simulink model "modelisation"  (R2018a)
settings: Solver=VariableStepAuto  StartTime=0.0  StopTime=10  RelTol=1e-3
values from neighbouring files (symbols this model uses):
  coderResolution = 370.0    (= 370)    [simu.m]
  D = xD + yD * 1i    [simu.m]
  dDirEcartMax = 5.0    (= 5)    [simu.m]
  dDirEcartMin = 1.0    (= 1)    [simu.m]
  distanceBetweenWheels = width    (= 250)    [simu.m]
  I = 0.0    (= 0)    [simu.m]
  motorNominalTension = 24.0    (= 24)    [simu.m]
  motorSpeedGain = (motorSpeedGainRPMpV / 60.0)    (= 3.88333333333)    [simu.m]
  oDirEcartMax = (45.0 / 360.0 * 2.0 * pi)    (= 0.785398163397)    [simu.m]
  oDirEcartMin = (6.0 / 360.0 * 2.0 * pi)    (= 0.10471975512)    [simu.m]
  oGain = 3.0    (= 3)    [simu.m]
  oinit = 4 * pi    (= 12.5663706144)    [simu.m]
  P = 3.0    (= 3)    [simu.m]
  reducRatio = (cranReducIn / cranReducOut)    (= 0.25)    [simu.m]
  wheelPerimeter = (wheelDiameter * pi)    (= 251.327412287)    [simu.m]
  xinit = 50    [simu.m]
  yinit = 50    [simu.m]
libraries: simulink x2
settings Model: Creator=geoffrey  LastModifiedBy=geoffrey
settings CodeAppCC: StateflowObjectComments=on

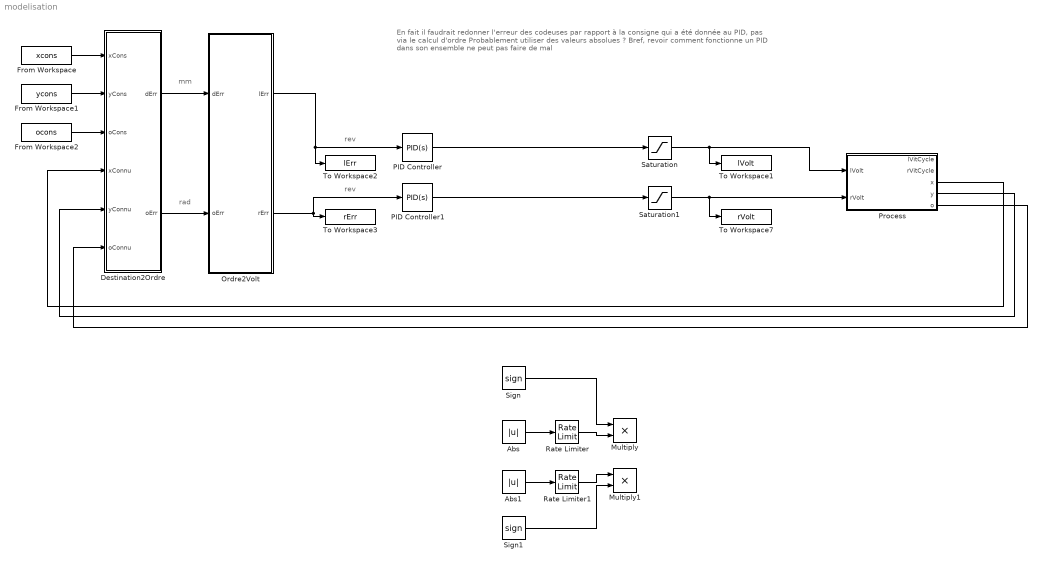
== system modelisation ==
  note: rev
  note: rad
  note: mm
  note: En fait il faudrait redonner l'erreur des codeuses par rapport à la consigne qui a été donnée au PID, pas via le calcul d'ordre
      | Probablement utiliser des valeurs absolues ?
      | Bref, revoir comment fonctionne un PID dans son ensemble ne peut pas faire de mal
  note: rev
  Abs : Abs
  Abs1 : Abs
  Destination2Ordre : Subsystem
  From Workspace : FromWorkspace  VariableName=xcons  SampleTime=0
  From Workspace1 : FromWorkspace  VariableName=ycons  SampleTime=0
  From Workspace2 : FromWorkspace  VariableName=ocons  SampleTime=0
  Multiply : Product
  Multiply1 : Product
  Ordre2Volt : Subsystem
  PID Controller : simulink/Continuous/PID Controller  Controller=PID  TimeDomain=Continuous-time  SampleTime=-1  IntegratorMethod=Forward Euler  FilterMethod=Forward Euler  Form=Parallel  UseFilter=on  ControllerParametersSource=internal  P=P  I=I  D=D  N=100  InitialConditionSource=internal  InitialConditionForIntegrator=0  InitialConditionForFilter=0  ExternalReset=none  LimitOutput=off  UpperSaturationLimit=inf  LowerSaturationLimit=-inf  LinearizeAsGain=on  AntiWindupMode=none  Kb=1  TrackingMode=off  Kt=1  PParamMin=[]  PParamMax=[]  IParamMin=[]  IParamMax=[]  DParamMin=[]  DParamMax=[]  NParamMin=[]  NParamMax=[]  KbParamMin=[]  KbParamMax=[]  KtParamMin=[]  KtParamMax=[]  POutMin=[]  POutMax=[]  IOutMin=[]  IOutMax=[]  DOutMin=[]  DOutMax=[]  NOutMin=[]  NOutMax=[]  KbOutMin=[]  KbOutMax=[]  KtOutMin=[]  KtOutMax=[]  IntegratorOutMin=[]  IntegratorOutMax=[]  FilterOutMin=[]  FilterOutMax=[]  SumOutMin=[]  SumOutMax=[]  SumI1OutMin=[]  SumI1OutMax=[]  SumI2OutMin=[]  SumI2OutMax=[]  SumI3OutMin=[]  SumI3OutMax=[]  SumDOutMin=[]  SumDOutMax=[]  SaturationOutMin=[]  SaturationOutMax=[]  IntegratorContinuousStateAttributes=''  IntegratorStateMustResolveToSignalObject=off  IntegratorRTWStateStorageClass=Auto  FilterContinuousStateAttributes=''  FilterStateMustResolveToSignalObject=off  FilterRTWStateStorageClass=Auto  DifferentiatorICPrevScaledInput=0  DifferentiatorOutMin=[]  DifferentiatorOutMax=[]  InitialConditionSetting=State (most efficient)  FilterDiffOutCoefMin=[]  FilterDiffOutCoefMax=[]  SumDenOutMin=[]  SumDenOutMax=[]  SumNumOutMin=[]  SumNumOutMax=[]  ReciprocalOutMin=[]  ReciprocalOutMax=[]  DivideOutMin=[]  DivideOutMax=[]  TunerSelectOption=Transfer Function Based (PID Tuner App)
  PID Controller1 : simulink/Continuous/PID Controller  Controller=PID  TimeDomain=Continuous-time  SampleTime=-1  IntegratorMethod=Forward Euler  FilterMethod=Forward Euler  Form=Parallel  UseFilter=on  ControllerParametersSource=internal  P=P  I=I  D=D  N=100  InitialConditionSource=internal  InitialConditionForIntegrator=0  InitialConditionForFilter=0  ExternalReset=none  LimitOutput=off  UpperSaturationLimit=inf  LowerSaturationLimit=-inf  LinearizeAsGain=on  AntiWindupMode=none  Kb=1  TrackingMode=off  Kt=1  PParamMin=[]  PParamMax=[]  IParamMin=[]  IParamMax=[]  DParamMin=[]  DParamMax=[]  NParamMin=[]  NParamMax=[]  KbParamMin=[]  KbParamMax=[]  KtParamMin=[]  KtParamMax=[]  POutMin=[]  POutMax=[]  IOutMin=[]  IOutMax=[]  DOutMin=[]  DOutMax=[]  NOutMin=[]  NOutMax=[]  KbOutMin=[]  KbOutMax=[]  KtOutMin=[]  KtOutMax=[]  IntegratorOutMin=[]  IntegratorOutMax=[]  FilterOutMin=[]  FilterOutMax=[]  SumOutMin=[]  SumOutMax=[]  SumI1OutMin=[]  SumI1OutMax=[]  SumI2OutMin=[]  SumI2OutMax=[]  SumI3OutMin=[]  SumI3OutMax=[]  SumDOutMin=[]  SumDOutMax=[]  SaturationOutMin=[]  SaturationOutMax=[]  IntegratorContinuousStateAttributes=''  IntegratorStateMustResolveToSignalObject=off  IntegratorRTWStateStorageClass=Auto  FilterContinuousStateAttributes=''  FilterStateMustResolveToSignalObject=off  FilterRTWStateStorageClass=Auto  DifferentiatorICPrevScaledInput=0  DifferentiatorOutMin=[]  DifferentiatorOutMax=[]  InitialConditionSetting=State (most efficient)  FilterDiffOutCoefMin=[]  FilterDiffOutCoefMax=[]  SumDenOutMin=[]  SumDenOutMax=[]  SumNumOutMin=[]  SumNumOutMax=[]  ReciprocalOutMin=[]  ReciprocalOutMax=[]  DivideOutMin=[]  DivideOutMax=[]  TunerSelectOption=Transfer Function Based (PID Tuner App)
  Process : Subsystem
  Rate Limiter : RateLimiter  FallingSlewLimit=-inf  SampleTimeMode=inherited
  Rate Limiter1 : RateLimiter  FallingSlewLimit=-inf  SampleTimeMode=inherited
  Saturation : Saturate  UpperLimit=motorNominalTension  LowerLimit=-motorNominalTension
  Saturation1 : Saturate  UpperLimit=motorNominalTension  LowerLimit=-motorNominalTension
  Sign : Signum
  Sign1 : Signum
  To Workspace1 : ToWorkspace  VariableName=lVolt  SaveFormat=Timeseries  SampleTime=-1
  To Workspace2 : ToWorkspace  VariableName=lErr  SaveFormat=Timeseries  SampleTime=-1
  To Workspace3 : ToWorkspace  VariableName=rErr  SaveFormat=Timeseries  SampleTime=-1
  To Workspace7 : ToWorkspace  VariableName=rVolt  SaveFormat=Timeseries  SampleTime=-1
  wires:
  Process/3(x) -> Destination2Ordre/4(xConnu)
  Process/4(y) -> Destination2Ordre/5(yConnu)
  Process/5(o) -> Destination2Ordre/6(oConnu)
  Saturation/1 -> To Workspace1/1, Process/1(lVolt)
  Saturation1/1 -> To Workspace7/1, Process/2(rVolt)
  From Workspace1/1 -> Destination2Ordre/2(yCons)
  From Workspace/1 -> Destination2Ordre/1(xCons)
  From Workspace2/1 -> Destination2Ordre/3(oCons)
  Ordre2Volt/1(lErr) -> To Workspace2/1, PID Controller/1
  Ordre2Volt/2(rErr) -> To Workspace3/1, PID Controller1/1
  Destination2Ordre/1(dErr) -> Ordre2Volt/1(dErr)
  Destination2Ordre/2(oErr) -> Ordre2Volt/2(oErr)
  PID Controller/1 -> Saturation/1
  PID Controller1/1 -> Saturation1/1
  Abs1/1 -> Rate Limiter1/1
  Sign1/1 -> Multiply1/2
  Rate Limiter/1 -> Multiply/2
  Rate Limiter1/1 -> Multiply1/1
  Abs/1 -> Rate Limiter/1
  ? -> Sign/1, Abs/1
  Sign/1 -> Multiply/1
  ? -> Sign1/1, Abs1/1

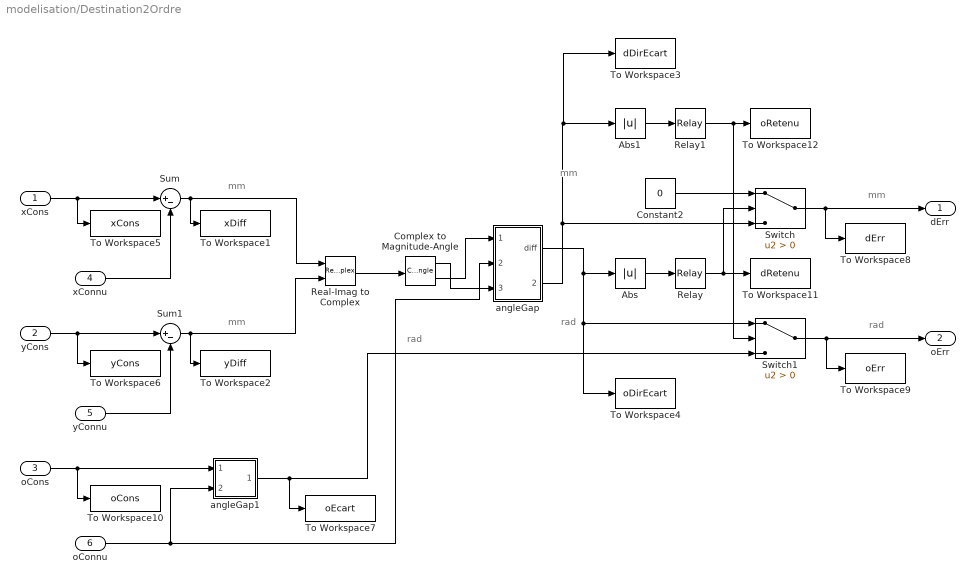
== system modelisation/Destination2Ordre ==
  note: mm
  note: rad
  note: rad
  note: mm
  note: rad
  note: mm
  note: mm
  xCons : Inport
  yCons : Inport  Port=2
  oCons : Inport  Port=3
  xConnu : Inport  Port=4
  yConnu : Inport  Port=5
  oConnu : Inport  Port=6
  Abs : Abs
  Abs1 : Abs
  Complex to Magnitude-Angle : ComplexToMagnitudeAngle
  Constant2 : Constant  Value=0
  Real-Imag to Complex : RealImagToComplex
  Relay : Relay  OnSwitchValue=oDirEcartMax  OffSwitchValue=oDirEcartMin
  Relay1 : Relay  OnSwitchValue=dDirEcartMax  OffSwitchValue=dDirEcartMin
  Sum : Sum  Inputs=|+-
  Sum1 : Sum  Inputs=|+-
  Switch : Switch  Criteria=u2 > Threshold
  Switch1 : Switch  Criteria=u2 > Threshold
  To Workspace1 : ToWorkspace  VariableName=xDiff  SaveFormat=Timeseries  SampleTime=-1
  To Workspace10 : ToWorkspace  VariableName=oCons  SaveFormat=Timeseries  SampleTime=-1
  To Workspace11 : ToWorkspace  VariableName=dRetenu  SaveFormat=Timeseries  SampleTime=-1
  To Workspace12 : ToWorkspace  VariableName=oRetenu  SaveFormat=Timeseries  SampleTime=-1
  To Workspace2 : ToWorkspace  VariableName=yDiff  SaveFormat=Timeseries  SampleTime=-1
  To Workspace3 : ToWorkspace  VariableName=dDirEcart  SaveFormat=Timeseries  SampleTime=-1
  To Workspace4 : ToWorkspace  VariableName=oDirEcart  SaveFormat=Timeseries  SampleTime=-1
  To Workspace5 : ToWorkspace  VariableName=xCons  SaveFormat=Timeseries  SampleTime=-1
  To Workspace6 : ToWorkspace  VariableName=yCons  SaveFormat=Timeseries  SampleTime=-1
  To Workspace7 : ToWorkspace  VariableName=oEcart  SaveFormat=Timeseries  SampleTime=-1
  To Workspace8 : ToWorkspace  VariableName=dErr  SaveFormat=Timeseries  SampleTime=-1
  To Workspace9 : ToWorkspace  VariableName=oErr  SaveFormat=Timeseries  SampleTime=-1
  angleGap : Subsystem
  angleGap1 : Subsystem
  dErr : Outport
  oErr : Outport  Port=2
  wires:
  xConnu/1 -> Sum/2
  xCons/1 -> Sum/1, To Workspace5/1
  Sum/1 -> Real-Imag to Complex/1, To Workspace1/1
  Sum1/1 -> Real-Imag to Complex/2, To Workspace2/1
  yConnu/1 -> Sum1/2
  Switch1/1 -> oErr/1, To Workspace9/1
  Switch/1 -> dErr/1, To Workspace8/1
  Real-Imag to Complex/1 -> Complex to Magnitude-Angle/1
  Relay/1 -> To Workspace11/1, Switch/2
  Constant2/1 -> Switch/1
  Relay1/1 -> To Workspace12/1, Switch1/2
  oConnu/1 -> angleGap1/2(actual), angleGap/2(actual)
  yCons/1 -> To Workspace6/1, Sum1/1
  oCons/1 -> angleGap1/1(target), To Workspace10/1
  Complex to Magnitude-Angle/2 -> angleGap/1(target)
  Abs/1 -> Relay/1
  angleGap/1(diff) -> Switch1/1, To Workspace4/1, Abs/1
  angleGap1/1(diff) -> To Workspace7/1, Switch1/3
  Complex to Magnitude-Angle/1 -> angleGap/3(dist)
  angleGap/2(distNew) -> To Workspace3/1, Abs1/1, Switch/3
  Abs1/1 -> Relay1/1

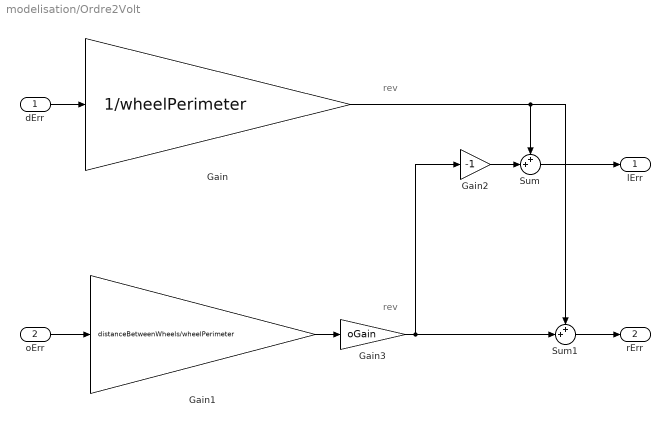
== system modelisation/Ordre2Volt ==
  note: rev
  note: rev
  dErr : Inport
  oErr : Inport  Port=2
  Gain : Gain  Gain=1/wheelPerimeter
  Gain1 : Gain  Gain=distanceBetweenWheels/wheelPerimeter
  Gain2 : Gain  Gain=-1
  Gain3 : Gain  Gain=oGain
  Sum : Sum  Inputs=++|
  Sum1 : Sum  Inputs=++|
  lErr : Outport
  rErr : Outport  Port=2
  wires:
  dErr/1 -> Gain/1
  Gain/1 -> Sum/1, Sum1/1
  oErr/1 -> Gain1/1
  Sum1/1 -> rErr/1
  Gain2/1 -> Sum/2
  Sum/1 -> lErr/1
  Gain1/1 -> Gain3/1
  Gain3/1 -> Gain2/1, Sum1/2

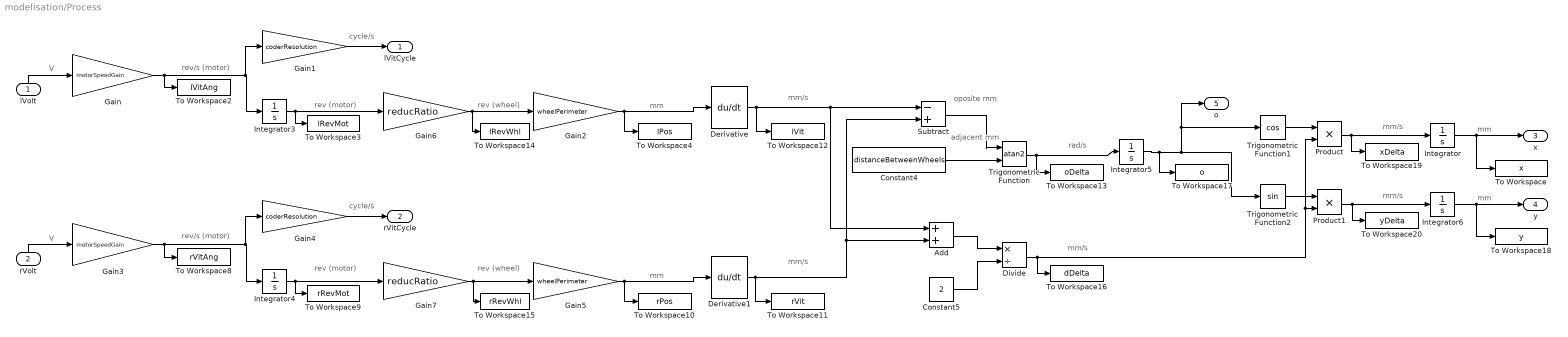
== system modelisation/Process ==
  note: mm
  note: mm/s
  note: rev (wheel)
  note: rad/s
  note: adjacent
      | mm
  note: oposite
      | mm
  note: mm/s
  note: mm/s
  note: mm
  note: rev (motor)
  note: cycle/s
  note: rev/s (motor)
  note: V
  note: mm
  note: cycle/s
  note: V
  note: rev (wheel)
  note: rev (motor)
  note: rev/s (motor)
  note: mm
  note: mm/s
  note: mm/s
  lVolt : Inport
  rVolt : Inport  Port=2
  Add : Sum
  Constant4 : Constant  Value=distanceBetweenWheels
  Constant5 : Constant  Value=2
  Derivative : Derivative
  Derivative1 : Derivative
  Divide : Product  Inputs=*/
  Gain : Gain  Gain=motorSpeedGain
  Gain1 : Gain  Gain=coderResolution
  Gain2 : Gain  Gain=wheelPerimeter
  Gain3 : Gain  Gain=motorSpeedGain
  Gain4 : Gain  Gain=coderResolution
  Gain5 : Gain  Gain=wheelPerimeter
  Gain6 : Gain  Gain=reducRatio
  Gain7 : Gain  Gain=reducRatio
  Integrator : Integrator  InitialCondition=xinit
  Integrator3 : Integrator
  Integrator4 : Integrator
  Integrator5 : Integrator  InitialCondition=oinit
  Integrator6 : Integrator  InitialCondition=yinit
  Product : Product
  Product1 : Product
  Subtract : Sum  Inputs=-+
  To Workspace : ToWorkspace  VariableName=x  SaveFormat=Timeseries  SampleTime=-1
  To Workspace10 : ToWorkspace  VariableName=rPos  SaveFormat=Timeseries  SampleTime=-1
  To Workspace11 : ToWorkspace  VariableName=rVit  SaveFormat=Timeseries  SampleTime=-1
  To Workspace12 : ToWorkspace  VariableName=lVit  SaveFormat=Timeseries  SampleTime=-1
  To Workspace13 : ToWorkspace  VariableName=oDelta  SaveFormat=Timeseries  SampleTime=-1
  To Workspace14 : ToWorkspace  VariableName=lRevWhl  SaveFormat=Timeseries  SampleTime=-1
  To Workspace15 : ToWorkspace  VariableName=rRevWhl  SaveFormat=Timeseries  SampleTime=-1
  To Workspace16 : ToWorkspace  VariableName=dDelta  SaveFormat=Timeseries  SampleTime=-1
  To Workspace17 : ToWorkspace  VariableName=o  SaveFormat=Timeseries  SampleTime=-1
  To Workspace18 : ToWorkspace  VariableName=y  SaveFormat=Timeseries  SampleTime=-1
  To Workspace19 : ToWorkspace  VariableName=xDelta  SaveFormat=Timeseries  SampleTime=-1
  To Workspace2 : ToWorkspace  VariableName=lVitAng  SaveFormat=Timeseries  SampleTime=-1
  To Workspace20 : ToWorkspace  VariableName=yDelta  SaveFormat=Timeseries  SampleTime=-1
  To Workspace3 : ToWorkspace  VariableName=lRevMot  SaveFormat=Timeseries  SampleTime=-1
  To Workspace4 : ToWorkspace  VariableName=lPos  SaveFormat=Timeseries  SampleTime=-1
  To Workspace8 : ToWorkspace  VariableName=rVitAng  SaveFormat=Timeseries  SampleTime=-1
  To Workspace9 : ToWorkspace  VariableName=rRevMot  SaveFormat=Timeseries  SampleTime=-1
  Trigonometric Function : Trigonometry  Operator=atan2
  Trigonometric Function1 : Trigonometry  Operator=cos
  Trigonometric Function2 : Trigonometry
  lVitCycle : Outport
  rVitCycle : Outport  Port=2
  x : Outport  Port=3
  y : Outport  Port=4
  o : Outport  Port=5
  wires:
  Derivative/1 -> To Workspace12/1, Add/1, Subtract/1
  Integrator/1 -> x/1, To Workspace/1
  Trigonometric Function1/1 -> Product/1
  Gain3/1 -> Gain4/1, Integrator4/1, To Workspace8/1
  Integrator5/1 -> Trigonometric Function2/1, o/1, Trigonometric Function1/1, To Workspace17/1
  Product/1 -> To Workspace19/1, Integrator/1
  Subtract/1 -> Trigonometric Function/1
  Gain2/1 -> Derivative/1, To Workspace4/1
  Gain5/1 -> Derivative1/1, To Workspace10/1
  Gain1/1 -> lVitCycle/1
  Gain/1 -> Gain1/1, Integrator3/1, To Workspace2/1
  Integrator3/1 -> Gain6/1, To Workspace3/1
  Constant5/1 -> Divide/2
  Add/1 -> Divide/1
  Gain7/1 -> To Workspace15/1, Gain5/1
  Derivative1/1 -> Add/2, Subtract/2, To Workspace11/1
  Gain4/1 -> rVitCycle/1
  Gain6/1 -> To Workspace14/1, Gain2/1
  Divide/1 -> Product1/2, Product/2, To Workspace16/1
  Trigonometric Function2/1 -> Product1/1
  lVolt/1 -> Gain/1
  rVolt/1 -> Gain3/1
  Constant4/1 -> Trigonometric Function/2
  Integrator6/1 -> y/1, To Workspace18/1
  Trigonometric Function/1 -> Integrator5/1, To Workspace13/1
  Integrator4/1 -> Gain7/1, To Workspace9/1
  Product1/1 -> To Workspace20/1, Integrator6/1

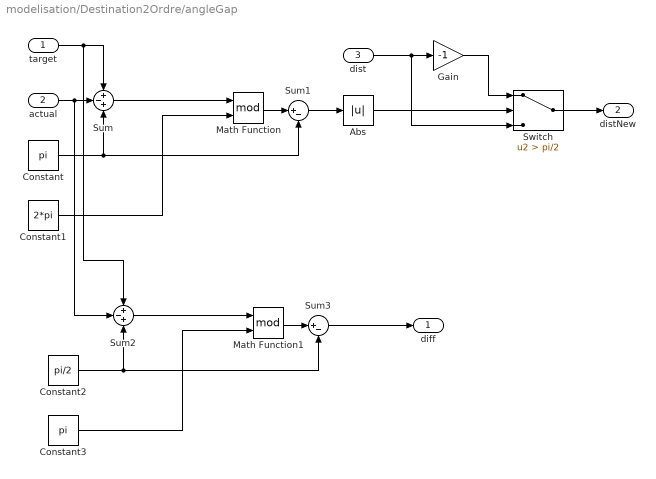
== system modelisation/Destination2Ordre/angleGap ==
  target : Inport
  actual : Inport  Port=2
  dist : Inport  Port=3
  Abs : Abs
  Constant : Constant  Value=pi
  Constant1 : Constant  Value=2*pi
  Constant2 : Constant  Value=pi/2
  Constant3 : Constant  Value=pi
  Gain : Gain  Gain=-1
  Math Function : Math  Operator=mod  SaturateOnIntegerOverflow=on
  Math Function1 : Math  Operator=mod  SaturateOnIntegerOverflow=on
  Sum : Sum  Inputs=+-+
  Sum1 : Sum  Inputs=|+-
  Sum2 : Sum  Inputs=+-+
  Sum3 : Sum  Inputs=|+-
  Switch : Switch  Criteria=u2 > Threshold  Threshold=pi/2
  diff : Outport
  distNew : Outport  Port=2
  wires:
  Sum/1 -> Math Function/1
  Math Function/1 -> Sum1/1
  Constant1/1 -> Math Function/2
  Constant/1 -> Sum1/2, Sum/3
  actual/1 -> Sum2/2, Sum/2
  target/1 -> Sum2/1, Sum/1
  Constant3/1 -> Math Function1/2
  Math Function1/1 -> Sum3/1
  Constant2/1 -> Sum3/2, Sum2/3
  Sum2/1 -> Math Function1/1
  Sum3/1 -> diff/1
  Sum1/1 -> Abs/1
  Abs/1 -> Switch/2
  dist/1 -> Gain/1, Switch/3
  Gain/1 -> Switch/1
  Switch/1 -> distNew/1

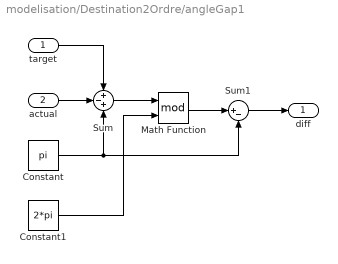
== system modelisation/Destination2Ordre/angleGap1 ==
  target : Inport
  actual : Inport  Port=2
  Constant : Constant  Value=pi
  Constant1 : Constant  Value=2*pi
  Math Function : Math  Operator=mod  SaturateOnIntegerOverflow=on
  Sum : Sum  Inputs=+-+
  Sum1 : Sum  Inputs=|+-
  diff : Outport
  wires:
  target/1 -> Sum/1
  Sum/1 -> Math Function/1
  Math Function/1 -> Sum1/1
  Sum1/1 -> diff/1
  Constant1/1 -> Math Function/2
  Constant/1 -> Sum1/2, Sum/3
  actual/1 -> Sum/2
